simulink library "debounce_lib_new"  (Simulink 8.1)
settings: Solver=ode45  StartTime=0.0  StopTime=10.0  RelTol=1e-3
undefined symbols (not defined in the file or in its folder): DiscIntNeverNeededParam
undefined symbols (not defined in the file): sampdT
libraries: simulink x1
settings Model: Creator=ch24070  LastModifiedBy=ch24070  CovSaveCumulativeToWorkspaceVar=on

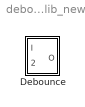
== system debounce_lib_new ==
  Debounce : Subsystem  mask{Ts=sampdT, Td=0.007}
      mask prompts: Ts "Sample Time"; Td "Debounce Time"

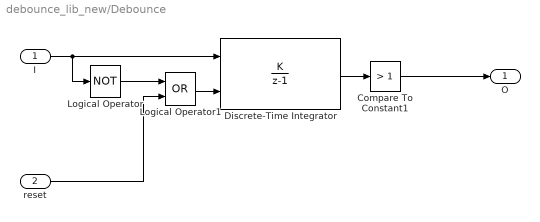
== system debounce_lib_new/Debounce ==
  I : Inport
  reset : Inport  Port=2
  Compare To Constant1 : simulink/Logic and Bit Operations/Compare To Constant  relop=>  const=1  OutDataTypeStr=boolean
  Discrete-Time Integrator : DiscreteIntegrator  IntegratorMethod=Accumulation: Forward Euler  gainval=Ts/Td  ExternalReset=level  SampleTime=Ts  OutDataTypeStr=fixdt(0,16,15)  LimitOutput=on  UpperSaturationLimit=1.001  LowerSaturationLimit=0  ICPrevOutput=DiscIntNeverNeededParam  ICPrevScaledInput=DiscIntNeverNeededParam
  Logical Operator : Logic  Operator=NOT  AllPortsSameDT=off  OutDataTypeStr=boolean
  Logical Operator1 : Logic  Operator=OR  AllPortsSameDT=off  OutDataTypeStr=boolean
  O : Outport
  wires:
  Discrete-Time Integrator/1 -> Compare To Constant1/1
  I/1 -> Discrete-Time Integrator/1, Logical Operator/1
  Compare To Constant1/1 -> O/1
  reset/1 -> Logical Operator1/2
  Logical Operator1/1 -> Discrete-Time Integrator/2
  Logical Operator/1 -> Logical Operator1/1
